simulink model "gm_parallel_prediction_and_cost_function_6phase"  (R2022a)
settings: Solver=FixedStepDiscrete  StartTime=0.0  StopTime=10.0  RelTol=1e-3
undefined symbols (not defined in the file or in its folder): f_c, L_d, L_q, L_x, L_y, p, psi_pm, R_ph
libraries: hdlmdlgenlib x338
(part 5 of 12)

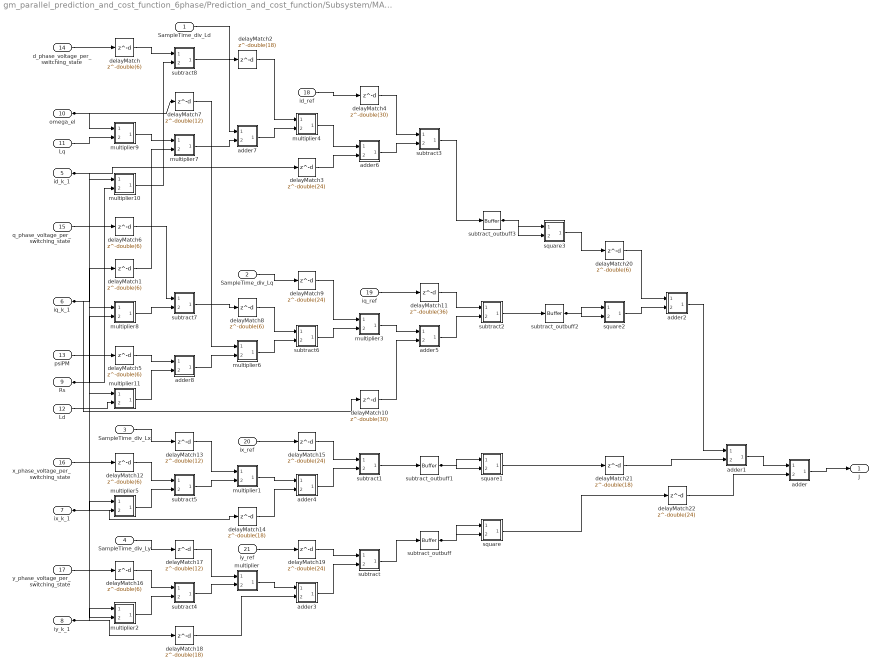
== system gm_parallel_prediction_and_cost_function_6phase/Prediction_and_cost_function/Subsystem/MATLAB Function ==
  SampleTime_div_Ld : Inport  OutDataTypeStr=single  PortDimensions=1  SampleTime=1e-08
  SampleTime_div_Lq : Inport  Port=2  OutDataTypeStr=single  PortDimensions=1  SampleTime=1e-08
  SampleTime_div_Lx : Inport  Port=3  OutDataTypeStr=single  PortDimensions=1  SampleTime=1e-08
  SampleTime_div_Ly : Inport  Port=4  OutDataTypeStr=single  PortDimensions=1  SampleTime=1e-08
  id_k_1 : Inport  Port=5  OutDataTypeStr=single  PortDimensions=1  SampleTime=1e-08
  iq_k_1 : Inport  Port=6  OutDataTypeStr=single  PortDimensions=1  SampleTime=1e-08
  ix_k_1 : Inport  Port=7  OutDataTypeStr=single  PortDimensions=1  SampleTime=1e-08
  iy_k_1 : Inport  Port=8  OutDataTypeStr=single  PortDimensions=1  SampleTime=1e-08
  Rs : Inport  Port=9  OutDataTypeStr=single  PortDimensions=1  SampleTime=1e-08
  omega_el : Inport  Port=10  OutDataTypeStr=single  PortDimensions=1  SampleTime=1e-08
  Lq : Inport  Port=11  OutDataTypeStr=single  PortDimensions=1  SampleTime=1e-08
  Ld : Inport  Port=12  OutDataTypeStr=single  PortDimensions=1  SampleTime=1e-08
  psiPM : Inport  Port=13  OutDataTypeStr=single  PortDimensions=1  SampleTime=1e-08
  d_phase_voltage_per_switching_state : Inport  Port=14  OutDataTypeStr=single  PortDimensions=1  SampleTime=1e-08
  q_phase_voltage_per_switching_state : Inport  Port=15  OutDataTypeStr=single  PortDimensions=1  SampleTime=1e-08
  x_phase_voltage_per_switching_state : Inport  Port=16  OutDataTypeStr=single  PortDimensions=1  SampleTime=1e-08
  y_phase_voltage_per_switching_state : Inport  Port=17  OutDataTypeStr=single  PortDimensions=1  SampleTime=1e-08
  id_ref : Inport  Port=18  OutDataTypeStr=single  PortDimensions=1  SampleTime=1e-08
  iq_ref : Inport  Port=19  OutDataTypeStr=single  PortDimensions=1  SampleTime=1e-08
  ix_ref : Inport  Port=20  OutDataTypeStr=single  PortDimensions=1  SampleTime=1e-08
  iy_ref : Inport  Port=21  OutDataTypeStr=single  PortDimensions=1  SampleTime=1e-08
  adder : Subsystem
      mask Display: disp('NFP\nadd');
  adder1 : Subsystem
      mask Display: disp('NFP\nadd');
  adder2 : Subsystem
      mask Display: disp('NFP\nadd');
  adder3 : Subsystem
      mask Display: disp('NFP\nadd');
  adder4 : Subsystem
      mask Display: disp('NFP\nadd');
  adder5 : Subsystem
      mask Display: disp('NFP\nadd');
  adder6 : Subsystem
      mask Display: disp('NFP\nadd');
  adder7 : Subsystem
      mask Display: disp('NFP\nadd');
  adder8 : Subsystem
      mask Display: disp('NFP\nadd');
  delayMatch{,1,5..6,8,12,16,20} (8 alike) : Delay  DelayLength=double(6)  InitialCondition=0  SampleTime=1e-08
  delayMatch10 : Delay  DelayLength=double(30)  InitialCondition=0  SampleTime=1e-08
  delayMatch11 : Delay  DelayLength=double(36)  InitialCondition=0  SampleTime=1e-08
  delayMatch13 : Delay  DelayLength=double(12)  InitialCondition=0  SampleTime=1e-08
  delayMatch{2,14,18,21} (4 alike) : Delay  DelayLength=double(18)  InitialCondition=0  SampleTime=1e-08
  delayMatch{3,9,15,19,22} (5 alike) : Delay  DelayLength=double(24)  InitialCondition=0  SampleTime=1e-08
  delayMatch17 : Delay  DelayLength=double(12)  InitialCondition=0  SampleTime=1e-08
  delayMatch4 : Delay  DelayLength=double(30)  InitialCondition=0  SampleTime=1e-08
  delayMatch7 : Delay  DelayLength=double(12)  InitialCondition=0  SampleTime=1e-08
  multiplier : Subsystem
      mask Display: disp('NFP\nmul');
  multiplier1 : Subsystem
      mask Display: disp('NFP\nmul');
  multiplier10 : Subsystem
      mask Display: disp('NFP\nmul');
  multiplier11 : Subsystem
      mask Display: disp('NFP\nmul');
  multiplier2 : Subsystem
      mask Display: disp('NFP\nmul');
  multiplier3 : Subsystem
      mask Display: disp('NFP\nmul');
  multiplier4 : Subsystem
      mask Display: disp('NFP\nmul');
  multiplier5 : Subsystem
      mask Display: disp('NFP\nmul');
  multiplier6 : Subsystem
      mask Display: disp('NFP\nmul');
  multiplier7 : Subsystem
      mask Display: disp('NFP\nmul');
  multiplier8 : Subsystem
      mask Display: disp('NFP\nmul');
  multiplier9 : Subsystem
      mask Display: disp('NFP\nmul');
  square : Subsystem
      mask Display: disp('NFP\nmul');
  square1 : Subsystem
      mask Display: disp('NFP\nmul');
  square2 : Subsystem
      mask Display: disp('NFP\nmul');
  square3 : Subsystem
      mask Display: disp('NFP\nmul');
  subtract : Subsystem
      mask Display: disp('NFP\nadd');
  subtract1 : Subsystem
      mask Display: disp('NFP\nadd');
  subtract2 : Subsystem
      mask Display: disp('NFP\nadd');
  subtract3 : Subsystem
      mask Display: disp('NFP\nadd');
  subtract4 : Subsystem
      mask Display: disp('NFP\nadd');
  subtract5 : Subsystem
      mask Display: disp('NFP\nadd');
  subtract6 : Subsystem
      mask Display: disp('NFP\nadd');
  subtract7 : Subsystem
      mask Display: disp('NFP\nadd');
  subtract8 : Subsystem
      mask Display: disp('NFP\nadd');
  subtract_outbuff{,1..3} (4 alike) : hdlmdlgenlib/Buffer
      settings: SourceProductBaseCode=SL
  J : Outport  SampleTime=1e-08  VectorParamsAs1DForOutWhenUnconnected=off
  wires:
  delayMatch2/1 -> multiplier4/1(In1)
  delayMatch9/1 -> multiplier3/1(In1)
  delayMatch13/1 -> multiplier1/1(In1)
  delayMatch17/1 -> multiplier/1(In1)
  delayMatch3/1 -> adder6/2(In2)
  delayMatch1/1 -> multiplier7/2(In2)
  delayMatch14/1 -> adder4/2(In2)
  delayMatch18/1 -> adder3/2(In2)
  delayMatch7/1 -> multiplier6/1(In1)
  delayMatch5/1 -> adder8/1(In1)
  delayMatch/1 -> subtract8/1(In1)
  delayMatch6/1 -> subtract7/1(In1)
  delayMatch12/1 -> subtract5/1(In1)
  delayMatch16/1 -> subtract4/1(In1)
  delayMatch4/1 -> subtract3/1(In1)
  delayMatch11/1 -> subtract2/1(In1)
  delayMatch15/1 -> subtract1/1(In1)
  delayMatch19/1 -> subtract/1(In1)
  delayMatch22/1 -> adder/2(In2)
  subtract_outbuff/1 -> square/2(In2), square/1(In1)
  delayMatch21/1 -> adder1/2(In2)
  subtract_outbuff1/1 -> square1/2(In2), square1/1(In1)
  delayMatch20/1 -> adder2/1(In1)
  subtract_outbuff2/1 -> square2/2(In2), square2/1(In1)
  subtract_outbuff3/1 -> square3/2(In2), square3/1(In1)
  delayMatch8/1 -> subtract6/1(In1)
  adder/1(Out1) -> J/1
  square/1(Out1) -> delayMatch22/1
  adder1/1(Out1) -> adder/1(In1)
  subtract/1(Out1) -> subtract_outbuff/1
  square1/1(Out1) -> delayMatch21/1
  adder2/1(Out1) -> adder1/1(In1)
  adder3/1(Out1) -> subtract/2(In2)
  subtract1/1(Out1) -> subtract_outbuff1/1
  square2/1(Out1) -> adder2/2(In2)
  square3/1(Out1) -> delayMatch20/1
  multiplier/1(Out1) -> adder3/1(In1)
  adder4/1(Out1) -> subtract1/2(In2)
  subtract2/1(Out1) -> subtract_outbuff2/1
  subtract3/1(Out1) -> subtract_outbuff3/1
  subtract4/1(Out1) -> multiplier/2(In2)
  multiplier1/1(Out1) -> adder4/1(In1)
  adder5/1(Out1) -> subtract2/2(In2)
  adder6/1(Out1) -> subtract3/2(In2)
  multiplier2/1(Out1) -> subtract4/2(In2)
  subtract5/1(Out1) -> multiplier1/2(In2)
  multiplier3/1(Out1) -> adder5/1(In1)
  multiplier4/1(Out1) -> adder6/1(In1)
  multiplier5/1(Out1) -> subtract5/2(In2)
  subtract6/1(Out1) -> multiplier3/2(In2)
  adder7/1(Out1) -> multiplier4/2(In2)
  multiplier6/1(Out1) -> subtract6/2(In2)
  subtract7/1(Out1) -> delayMatch8/1
  multiplier7/1(Out1) -> adder7/2(In2)
  subtract8/1(Out1) -> adder7/1(In1)
  adder8/1(Out1) -> multiplier6/2(In2)
  multiplier8/1(Out1) -> subtract7/2(In2)
  multiplier9/1(Out1) -> multiplier7/1(In1)
  multiplier10/1(Out1) -> subtract8/2(In2)
  multiplier11/1(Out1) -> adder8/2(In2)
  delayMatch10/1 -> adder5/2(In2)
  SampleTime_div_Ld/1 -> delayMatch2/1
  SampleTime_div_Lq/1 -> delayMatch9/1
  SampleTime_div_Lx/1 -> delayMatch13/1
  SampleTime_div_Ly/1 -> delayMatch17/1
  id_k_1/1 -> delayMatch3/1, multiplier11/1(In1), multiplier10/1(In1)
  iq_k_1/1 -> delayMatch10/1, delayMatch1/1, multiplier8/1(In1)
  ix_k_1/1 -> delayMatch14/1, multiplier5/1(In1)
  iy_k_1/1 -> delayMatch18/1, multiplier2/1(In1)
  Rs/1 -> multiplier10/2(In2), multiplier8/2(In2), multiplier5/2(In2), multiplier2/2(In2)
  omega_el/1 -> delayMatch7/1, multiplier9/1(In1)
  Lq/1 -> multiplier9/2(In2)
  Ld/1 -> multiplier11/2(In2)
  psiPM/1 -> delayMatch5/1
  d_phase_voltage_per_switching_state/1 -> delayMatch/1
  q_phase_voltage_per_switching_state/1 -> delayMatch6/1
  x_phase_voltage_per_switching_state/1 -> delayMatch12/1
  y_phase_voltage_per_switching_state/1 -> delayMatch16/1
  id_ref/1 -> delayMatch4/1
  iq_ref/1 -> delayMatch11/1
  ix_ref/1 -> delayMatch15/1
  iy_ref/1 -> delayMatch19/1

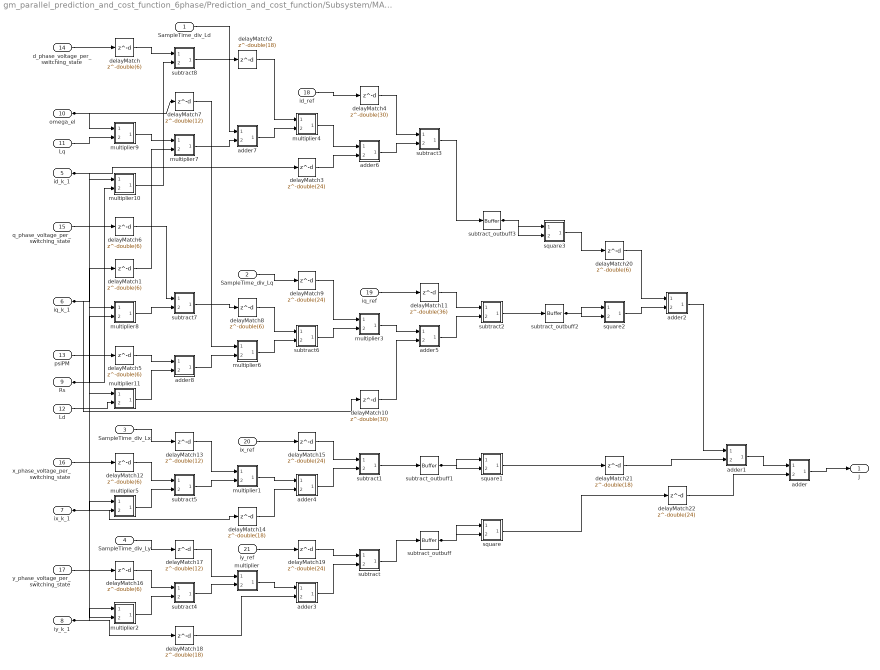
== system gm_parallel_prediction_and_cost_function_6phase/Prediction_and_cost_function/Subsystem/MATLAB Function1 ==
  SampleTime_div_Ld : Inport  OutDataTypeStr=single  PortDimensions=1  SampleTime=1e-08
  SampleTime_div_Lq : Inport  Port=2  OutDataTypeStr=single  PortDimensions=1  SampleTime=1e-08
  SampleTime_div_Lx : Inport  Port=3  OutDataTypeStr=single  PortDimensions=1  SampleTime=1e-08
  SampleTime_div_Ly : Inport  Port=4  OutDataTypeStr=single  PortDimensions=1  SampleTime=1e-08
  id_k_1 : Inport  Port=5  OutDataTypeStr=single  PortDimensions=1  SampleTime=1e-08
  iq_k_1 : Inport  Port=6  OutDataTypeStr=single  PortDimensions=1  SampleTime=1e-08
  ix_k_1 : Inport  Port=7  OutDataTypeStr=single  PortDimensions=1  SampleTime=1e-08
  iy_k_1 : Inport  Port=8  OutDataTypeStr=single  PortDimensions=1  SampleTime=1e-08
  Rs : Inport  Port=9  OutDataTypeStr=single  PortDimensions=1  SampleTime=1e-08
  omega_el : Inport  Port=10  OutDataTypeStr=single  PortDimensions=1  SampleTime=1e-08
  Lq : Inport  Port=11  OutDataTypeStr=single  PortDimensions=1  SampleTime=1e-08
  Ld : Inport  Port=12  OutDataTypeStr=single  PortDimensions=1  SampleTime=1e-08
  psiPM : Inport  Port=13  OutDataTypeStr=single  PortDimensions=1  SampleTime=1e-08
  d_phase_voltage_per_switching_state : Inport  Port=14  OutDataTypeStr=single  PortDimensions=1  SampleTime=1e-08
  q_phase_voltage_per_switching_state : Inport  Port=15  OutDataTypeStr=single  PortDimensions=1  SampleTime=1e-08
  x_phase_voltage_per_switching_state : Inport  Port=16  OutDataTypeStr=single  PortDimensions=1  SampleTime=1e-08
  y_phase_voltage_per_switching_state : Inport  Port=17  OutDataTypeStr=single  PortDimensions=1  SampleTime=1e-08
  id_ref : Inport  Port=18  OutDataTypeStr=single  PortDimensions=1  SampleTime=1e-08
  iq_ref : Inport  Port=19  OutDataTypeStr=single  PortDimensions=1  SampleTime=1e-08
  ix_ref : Inport  Port=20  OutDataTypeStr=single  PortDimensions=1  SampleTime=1e-08
  iy_ref : Inport  Port=21  OutDataTypeStr=single  PortDimensions=1  SampleTime=1e-08
  adder : Subsystem
      mask Display: disp('NFP\nadd');
  adder1 : Subsystem
      mask Display: disp('NFP\nadd');
  adder2 : Subsystem
      mask Display: disp('NFP\nadd');
  adder3 : Subsystem
      mask Display: disp('NFP\nadd');
  adder4 : Subsystem
      mask Display: disp('NFP\nadd');
  adder5 : Subsystem
      mask Display: disp('NFP\nadd');
  adder6 : Subsystem
      mask Display: disp('NFP\nadd');
  adder7 : Subsystem
      mask Display: disp('NFP\nadd');
  adder8 : Subsystem
      mask Display: disp('NFP\nadd');
  delayMatch{,1,5..6,8,12,16,20} (8 alike) : Delay  DelayLength=double(6)  InitialCondition=0  SampleTime=1e-08
  delayMatch10 : Delay  DelayLength=double(30)  InitialCondition=0  SampleTime=1e-08
  delayMatch11 : Delay  DelayLength=double(36)  InitialCondition=0  SampleTime=1e-08
  delayMatch13 : Delay  DelayLength=double(12)  InitialCondition=0  SampleTime=1e-08
  delayMatch{2,14,18,21} (4 alike) : Delay  DelayLength=double(18)  InitialCondition=0  SampleTime=1e-08
  delayMatch{3,9,15,19,22} (5 alike) : Delay  DelayLength=double(24)  InitialCondition=0  SampleTime=1e-08
  delayMatch17 : Delay  DelayLength=double(12)  InitialCondition=0  SampleTime=1e-08
  delayMatch4 : Delay  DelayLength=double(30)  InitialCondition=0  SampleTime=1e-08
  delayMatch7 : Delay  DelayLength=double(12)  InitialCondition=0  SampleTime=1e-08
  multiplier : Subsystem
      mask Display: disp('NFP\nmul');
  multiplier1 : Subsystem
      mask Display: disp('NFP\nmul');
  multiplier10 : Subsystem
      mask Display: disp('NFP\nmul');
  multiplier11 : Subsystem
      mask Display: disp('NFP\nmul');
  multiplier2 : Subsystem
      mask Display: disp('NFP\nmul');
  multiplier3 : Subsystem
      mask Display: disp('NFP\nmul');
  multiplier4 : Subsystem
      mask Display: disp('NFP\nmul');
  multiplier5 : Subsystem
      mask Display: disp('NFP\nmul');
  multiplier6 : Subsystem
      mask Display: disp('NFP\nmul');
  multiplier7 : Subsystem
      mask Display: disp('NFP\nmul');
  multiplier8 : Subsystem
      mask Display: disp('NFP\nmul');
  multiplier9 : Subsystem
      mask Display: disp('NFP\nmul');
  square : Subsystem
      mask Display: disp('NFP\nmul');
  square1 : Subsystem
      mask Display: disp('NFP\nmul');
  square2 : Subsystem
      mask Display: disp('NFP\nmul');
  square3 : Subsystem
      mask Display: disp('NFP\nmul');
  subtract : Subsystem
      mask Display: disp('NFP\nadd');
  subtract1 : Subsystem
      mask Display: disp('NFP\nadd');
  subtract2 : Subsystem
      mask Display: disp('NFP\nadd');
  subtract3 : Subsystem
      mask Display: disp('NFP\nadd');
  subtract4 : Subsystem
      mask Display: disp('NFP\nadd');
  subtract5 : Subsystem
      mask Display: disp('NFP\nadd');
  subtract6 : Subsystem
      mask Display: disp('NFP\nadd');
  subtract7 : Subsystem
      mask Display: disp('NFP\nadd');
  subtract8 : Subsystem
      mask Display: disp('NFP\nadd');
  subtract_outbuff{,1..3} (4 alike) : hdlmdlgenlib/Buffer
      settings: SourceProductBaseCode=SL
  J : Outport  SampleTime=1e-08  VectorParamsAs1DForOutWhenUnconnected=off
  wires:
  iy_ref/1 -> delayMatch19/1
  ix_ref/1 -> delayMatch15/1
  iq_ref/1 -> delayMatch11/1
  id_ref/1 -> delayMatch4/1
  y_phase_voltage_per_switching_state/1 -> delayMatch16/1
  x_phase_voltage_per_switching_state/1 -> delayMatch12/1
  q_phase_voltage_per_switching_state/1 -> delayMatch6/1
  d_phase_voltage_per_switching_state/1 -> delayMatch/1
  psiPM/1 -> delayMatch5/1
  Ld/1 -> multiplier11/2(In2)
  Lq/1 -> multiplier9/2(In2)
  omega_el/1 -> multiplier9/1(In1), delayMatch7/1
  Rs/1 -> multiplier2/2(In2), multiplier5/2(In2), multiplier8/2(In2), multiplier10/2(In2)
  iy_k_1/1 -> multiplier2/1(In1), delayMatch18/1
  ix_k_1/1 -> multiplier5/1(In1), delayMatch14/1
  iq_k_1/1 -> multiplier8/1(In1), delayMatch1/1, delayMatch10/1
  id_k_1/1 -> multiplier10/1(In1), multiplier11/1(In1), delayMatch3/1
  SampleTime_div_Ly/1 -> delayMatch17/1
  SampleTime_div_Lx/1 -> delayMatch13/1
  SampleTime_div_Lq/1 -> delayMatch9/1
  SampleTime_div_Ld/1 -> delayMatch2/1
  delayMatch10/1 -> adder5/2(In2)
  multiplier11/1(Out1) -> adder8/2(In2)
  multiplier10/1(Out1) -> subtract8/2(In2)
  multiplier9/1(Out1) -> multiplier7/1(In1)
  multiplier8/1(Out1) -> subtract7/2(In2)
  adder8/1(Out1) -> multiplier6/2(In2)
  subtract8/1(Out1) -> adder7/1(In1)
  multiplier7/1(Out1) -> adder7/2(In2)
  subtract7/1(Out1) -> delayMatch8/1
  multiplier6/1(Out1) -> subtract6/2(In2)
  adder7/1(Out1) -> multiplier4/2(In2)
  subtract6/1(Out1) -> multiplier3/2(In2)
  multiplier5/1(Out1) -> subtract5/2(In2)
  multiplier4/1(Out1) -> adder6/1(In1)
  multiplier3/1(Out1) -> adder5/1(In1)
  subtract5/1(Out1) -> multiplier1/2(In2)
  multiplier2/1(Out1) -> subtract4/2(In2)
  adder6/1(Out1) -> subtract3/2(In2)
  adder5/1(Out1) -> subtract2/2(In2)
  multiplier1/1(Out1) -> adder4/1(In1)
  subtract4/1(Out1) -> multiplier/2(In2)
  subtract3/1(Out1) -> subtract_outbuff3/1
  subtract2/1(Out1) -> subtract_outbuff2/1
  adder4/1(Out1) -> subtract1/2(In2)
  multiplier/1(Out1) -> adder3/1(In1)
  square3/1(Out1) -> delayMatch20/1
  square2/1(Out1) -> adder2/2(In2)
  subtract1/1(Out1) -> subtract_outbuff1/1
  adder3/1(Out1) -> subtract/2(In2)
  adder2/1(Out1) -> adder1/1(In1)
  square1/1(Out1) -> delayMatch21/1
  subtract/1(Out1) -> subtract_outbuff/1
  adder1/1(Out1) -> adder/1(In1)
  square/1(Out1) -> delayMatch22/1
  adder/1(Out1) -> J/1
  delayMatch8/1 -> subtract6/1(In1)
  subtract_outbuff3/1 -> square3/1(In1), square3/2(In2)
  subtract_outbuff2/1 -> square2/1(In1), square2/2(In2)
  delayMatch20/1 -> adder2/1(In1)
  subtract_outbuff1/1 -> square1/1(In1), square1/2(In2)
  delayMatch21/1 -> adder1/2(In2)
  subtract_outbuff/1 -> square/1(In1), square/2(In2)
  delayMatch22/1 -> adder/2(In2)
  delayMatch19/1 -> subtract/1(In1)
  delayMatch15/1 -> subtract1/1(In1)
  delayMatch11/1 -> subtract2/1(In1)
  delayMatch4/1 -> subtract3/1(In1)
  delayMatch16/1 -> subtract4/1(In1)
  delayMatch12/1 -> subtract5/1(In1)
  delayMatch6/1 -> subtract7/1(In1)
  delayMatch/1 -> subtract8/1(In1)
  delayMatch5/1 -> adder8/1(In1)
  delayMatch7/1 -> multiplier6/1(In1)
  delayMatch18/1 -> adder3/2(In2)
  delayMatch14/1 -> adder4/2(In2)
  delayMatch1/1 -> multiplier7/2(In2)
  delayMatch3/1 -> adder6/2(In2)
  delayMatch17/1 -> multiplier/1(In1)
  delayMatch13/1 -> multiplier1/1(In1)
  delayMatch9/1 -> multiplier3/1(In1)
  delayMatch2/1 -> multiplier4/1(In1)

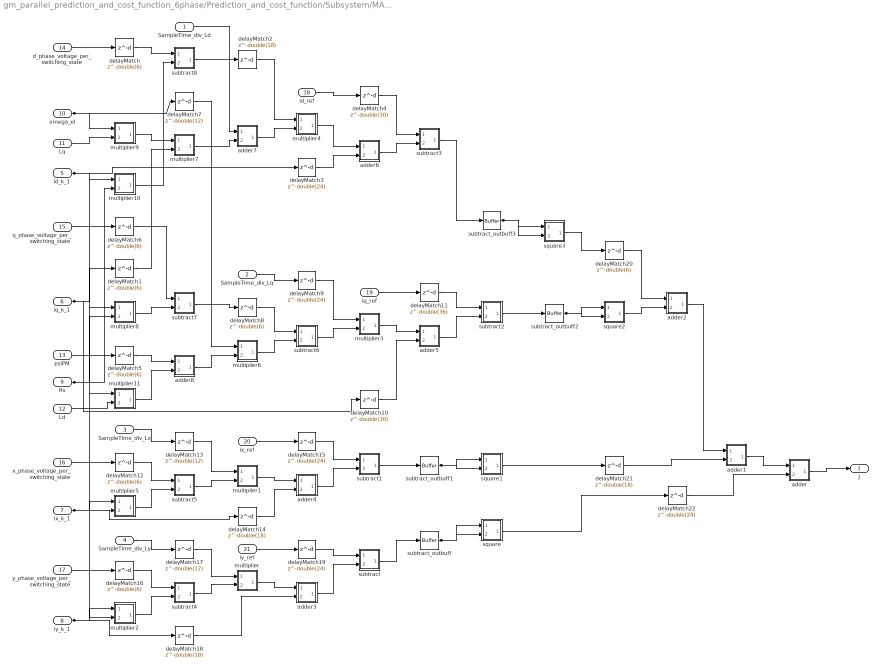
== system gm_parallel_prediction_and_cost_function_6phase/Prediction_and_cost_function/Subsystem/MATLAB Function10 ==
  SampleTime_div_Ld : Inport  OutDataTypeStr=single  PortDimensions=1  SampleTime=1e-08
  SampleTime_div_Lq : Inport  Port=2  OutDataTypeStr=single  PortDimensions=1  SampleTime=1e-08
  SampleTime_div_Lx : Inport  Port=3  OutDataTypeStr=single  PortDimensions=1  SampleTime=1e-08
  SampleTime_div_Ly : Inport  Port=4  OutDataTypeStr=single  PortDimensions=1  SampleTime=1e-08
  id_k_1 : Inport  Port=5  OutDataTypeStr=single  PortDimensions=1  SampleTime=1e-08
  iq_k_1 : Inport  Port=6  OutDataTypeStr=single  PortDimensions=1  SampleTime=1e-08
  ix_k_1 : Inport  Port=7  OutDataTypeStr=single  PortDimensions=1  SampleTime=1e-08
  iy_k_1 : Inport  Port=8  OutDataTypeStr=single  PortDimensions=1  SampleTime=1e-08
  Rs : Inport  Port=9  OutDataTypeStr=single  PortDimensions=1  SampleTime=1e-08
  omega_el : Inport  Port=10  OutDataTypeStr=single  PortDimensions=1  SampleTime=1e-08
  Lq : Inport  Port=11  OutDataTypeStr=single  PortDimensions=1  SampleTime=1e-08
  Ld : Inport  Port=12  OutDataTypeStr=single  PortDimensions=1  SampleTime=1e-08
  psiPM : Inport  Port=13  OutDataTypeStr=single  PortDimensions=1  SampleTime=1e-08
  d_phase_voltage_per_switching_state : Inport  Port=14  OutDataTypeStr=single  PortDimensions=1  SampleTime=1e-08
  q_phase_voltage_per_switching_state : Inport  Port=15  OutDataTypeStr=single  PortDimensions=1  SampleTime=1e-08
  x_phase_voltage_per_switching_state : Inport  Port=16  OutDataTypeStr=single  PortDimensions=1  SampleTime=1e-08
  y_phase_voltage_per_switching_state : Inport  Port=17  OutDataTypeStr=single  PortDimensions=1  SampleTime=1e-08
  id_ref : Inport  Port=18  OutDataTypeStr=single  PortDimensions=1  SampleTime=1e-08
  iq_ref : Inport  Port=19  OutDataTypeStr=single  PortDimensions=1  SampleTime=1e-08
  ix_ref : Inport  Port=20  OutDataTypeStr=single  PortDimensions=1  SampleTime=1e-08
  iy_ref : Inport  Port=21  OutDataTypeStr=single  PortDimensions=1  SampleTime=1e-08
  adder : Subsystem
      mask Display: disp('NFP\nadd');
  adder1 : Subsystem
      mask Display: disp('NFP\nadd');
  adder2 : Subsystem
      mask Display: disp('NFP\nadd');
  adder3 : Subsystem
      mask Display: disp('NFP\nadd');
  adder4 : Subsystem
      mask Display: disp('NFP\nadd');
  adder5 : Subsystem
      mask Display: disp('NFP\nadd');
  adder6 : Subsystem
      mask Display: disp('NFP\nadd');
  adder7 : Subsystem
      mask Display: disp('NFP\nadd');
  adder8 : Subsystem
      mask Display: disp('NFP\nadd');
  delayMatch{,1,5..6,8,12,16,20} (8 alike) : Delay  DelayLength=double(6)  InitialCondition=0  SampleTime=1e-08
  delayMatch10 : Delay  DelayLength=double(30)  InitialCondition=0  SampleTime=1e-08
  delayMatch11 : Delay  DelayLength=double(36)  InitialCondition=0  SampleTime=1e-08
  delayMatch13 : Delay  DelayLength=double(12)  InitialCondition=0  SampleTime=1e-08
  delayMatch{2,14,18,21} (4 alike) : Delay  DelayLength=double(18)  InitialCondition=0  SampleTime=1e-08
  delayMatch{3,9,15,19,22} (5 alike) : Delay  DelayLength=double(24)  InitialCondition=0  SampleTime=1e-08
  delayMatch17 : Delay  DelayLength=double(12)  InitialCondition=0  SampleTime=1e-08
  delayMatch4 : Delay  DelayLength=double(30)  InitialCondition=0  SampleTime=1e-08
  delayMatch7 : Delay  DelayLength=double(12)  InitialCondition=0  SampleTime=1e-08
  multiplier : Subsystem
      mask Display: disp('NFP\nmul');
  multiplier1 : Subsystem
      mask Display: disp('NFP\nmul');
  multiplier10 : Subsystem
      mask Display: disp('NFP\nmul');
  multiplier11 : Subsystem
      mask Display: disp('NFP\nmul');
  multiplier2 : Subsystem
      mask Display: disp('NFP\nmul');
  multiplier3 : Subsystem
      mask Display: disp('NFP\nmul');
  multiplier4 : Subsystem
      mask Display: disp('NFP\nmul');
  multiplier5 : Subsystem
      mask Display: disp('NFP\nmul');
  multiplier6 : Subsystem
      mask Display: disp('NFP\nmul');
  multiplier7 : Subsystem
      mask Display: disp('NFP\nmul');
  multiplier8 : Subsystem
      mask Display: disp('NFP\nmul');
  multiplier9 : Subsystem
      mask Display: disp('NFP\nmul');
  square : Subsystem
      mask Display: disp('NFP\nmul');
  square1 : Subsystem
      mask Display: disp('NFP\nmul');
  square2 : Subsystem
      mask Display: disp('NFP\nmul');
  square3 : Subsystem
      mask Display: disp('NFP\nmul');
  subtract : Subsystem
      mask Display: disp('NFP\nadd');
  subtract1 : Subsystem
      mask Display: disp('NFP\nadd');
  subtract2 : Subsystem
      mask Display: disp('NFP\nadd');
  subtract3 : Subsystem
      mask Display: disp('NFP\nadd');
  subtract4 : Subsystem
      mask Display: disp('NFP\nadd');
  subtract5 : Subsystem
      mask Display: disp('NFP\nadd');
  subtract6 : Subsystem
      mask Display: disp('NFP\nadd');
  subtract7 : Subsystem
      mask Display: disp('NFP\nadd');
  subtract8 : Subsystem
      mask Display: disp('NFP\nadd');
  subtract_outbuff{,1..3} (4 alike) : hdlmdlgenlib/Buffer
      settings: SourceProductBaseCode=SL
  J : Outport  SampleTime=1e-08  VectorParamsAs1DForOutWhenUnconnected=off
  wires:
  iy_ref/1 -> delayMatch19/1
  ix_ref/1 -> delayMatch15/1
  iq_ref/1 -> delayMatch11/1
  id_ref/1 -> delayMatch4/1
  y_phase_voltage_per_switching_state/1 -> delayMatch16/1
  x_phase_voltage_per_switching_state/1 -> delayMatch12/1
  q_phase_voltage_per_switching_state/1 -> delayMatch6/1
  d_phase_voltage_per_switching_state/1 -> delayMatch/1
  psiPM/1 -> delayMatch5/1
  Ld/1 -> multiplier11/2(In2)
  Lq/1 -> multiplier9/2(In2)
  omega_el/1 -> multiplier9/1(In1), delayMatch7/1
  Rs/1 -> multiplier2/2(In2), multiplier5/2(In2), multiplier8/2(In2), multiplier10/2(In2)
  iy_k_1/1 -> multiplier2/1(In1), delayMatch18/1
  ix_k_1/1 -> multiplier5/1(In1), delayMatch14/1
  iq_k_1/1 -> multiplier8/1(In1), delayMatch1/1, delayMatch10/1
  id_k_1/1 -> multiplier10/1(In1), multiplier11/1(In1), delayMatch3/1
  SampleTime_div_Ly/1 -> delayMatch17/1
  SampleTime_div_Lx/1 -> delayMatch13/1
  SampleTime_div_Lq/1 -> delayMatch9/1
  SampleTime_div_Ld/1 -> delayMatch2/1
  delayMatch10/1 -> adder5/2(In2)
  multiplier11/1(Out1) -> adder8/2(In2)
  multiplier10/1(Out1) -> subtract8/2(In2)
  multiplier9/1(Out1) -> multiplier7/1(In1)
  multiplier8/1(Out1) -> subtract7/2(In2)
  adder8/1(Out1) -> multiplier6/2(In2)
  subtract8/1(Out1) -> adder7/1(In1)
  multiplier7/1(Out1) -> adder7/2(In2)
  subtract7/1(Out1) -> delayMatch8/1
  multiplier6/1(Out1) -> subtract6/2(In2)
  adder7/1(Out1) -> multiplier4/2(In2)
  subtract6/1(Out1) -> multiplier3/2(In2)
  multiplier5/1(Out1) -> subtract5/2(In2)
  multiplier4/1(Out1) -> adder6/1(In1)
  multiplier3/1(Out1) -> adder5/1(In1)
  subtract5/1(Out1) -> multiplier1/2(In2)
  multiplier2/1(Out1) -> subtract4/2(In2)
  adder6/1(Out1) -> subtract3/2(In2)
  adder5/1(Out1) -> subtract2/2(In2)
  multiplier1/1(Out1) -> adder4/1(In1)
  subtract4/1(Out1) -> multiplier/2(In2)
  subtract3/1(Out1) -> subtract_outbuff3/1
  subtract2/1(Out1) -> subtract_outbuff2/1
  adder4/1(Out1) -> subtract1/2(In2)
  multiplier/1(Out1) -> adder3/1(In1)
  square3/1(Out1) -> delayMatch20/1
  square2/1(Out1) -> adder2/2(In2)
  subtract1/1(Out1) -> subtract_outbuff1/1
  adder3/1(Out1) -> subtract/2(In2)
  adder2/1(Out1) -> adder1/1(In1)
  square1/1(Out1) -> delayMatch21/1
  subtract/1(Out1) -> subtract_outbuff/1
  adder1/1(Out1) -> adder/1(In1)
  square/1(Out1) -> delayMatch22/1
  adder/1(Out1) -> J/1
  delayMatch8/1 -> subtract6/1(In1)
  subtract_outbuff3/1 -> square3/1(In1), square3/2(In2)
  subtract_outbuff2/1 -> square2/1(In1), square2/2(In2)
  delayMatch20/1 -> adder2/1(In1)
  subtract_outbuff1/1 -> square1/1(In1), square1/2(In2)
  delayMatch21/1 -> adder1/2(In2)
  subtract_outbuff/1 -> square/1(In1), square/2(In2)
  delayMatch22/1 -> adder/2(In2)
  delayMatch19/1 -> subtract/1(In1)
  delayMatch15/1 -> subtract1/1(In1)
  delayMatch11/1 -> subtract2/1(In1)
  delayMatch4/1 -> subtract3/1(In1)
  delayMatch16/1 -> subtract4/1(In1)
  delayMatch12/1 -> subtract5/1(In1)
  delayMatch6/1 -> subtract7/1(In1)
  delayMatch/1 -> subtract8/1(In1)
  delayMatch5/1 -> adder8/1(In1)
  delayMatch7/1 -> multiplier6/1(In1)
  delayMatch18/1 -> adder3/2(In2)
  delayMatch14/1 -> adder4/2(In2)
  delayMatch1/1 -> multiplier7/2(In2)
  delayMatch3/1 -> adder6/2(In2)
  delayMatch17/1 -> multiplier/1(In1)
  delayMatch13/1 -> multiplier1/1(In1)
  delayMatch9/1 -> multiplier3/1(In1)
  delayMatch2/1 -> multiplier4/1(In1)

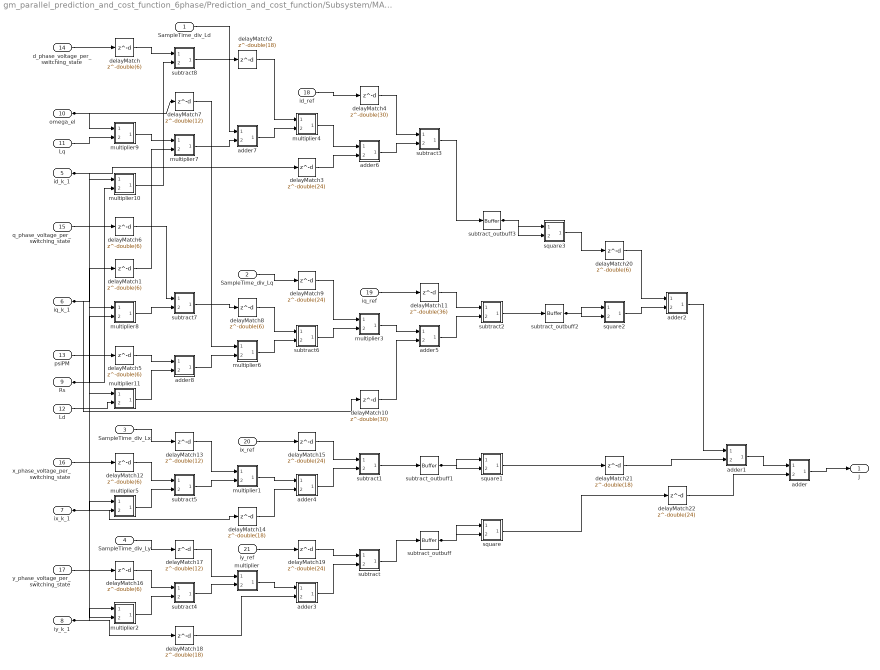
== system gm_parallel_prediction_and_cost_function_6phase/Prediction_and_cost_function/Subsystem/MATLAB Function11 ==
  SampleTime_div_Ld : Inport  OutDataTypeStr=single  PortDimensions=1  SampleTime=1e-08
  SampleTime_div_Lq : Inport  Port=2  OutDataTypeStr=single  PortDimensions=1  SampleTime=1e-08
  SampleTime_div_Lx : Inport  Port=3  OutDataTypeStr=single  PortDimensions=1  SampleTime=1e-08
  SampleTime_div_Ly : Inport  Port=4  OutDataTypeStr=single  PortDimensions=1  SampleTime=1e-08
  id_k_1 : Inport  Port=5  OutDataTypeStr=single  PortDimensions=1  SampleTime=1e-08
  iq_k_1 : Inport  Port=6  OutDataTypeStr=single  PortDimensions=1  SampleTime=1e-08
  ix_k_1 : Inport  Port=7  OutDataTypeStr=single  PortDimensions=1  SampleTime=1e-08
  iy_k_1 : Inport  Port=8  OutDataTypeStr=single  PortDimensions=1  SampleTime=1e-08
  Rs : Inport  Port=9  OutDataTypeStr=single  PortDimensions=1  SampleTime=1e-08
  omega_el : Inport  Port=10  OutDataTypeStr=single  PortDimensions=1  SampleTime=1e-08
  Lq : Inport  Port=11  OutDataTypeStr=single  PortDimensions=1  SampleTime=1e-08
  Ld : Inport  Port=12  OutDataTypeStr=single  PortDimensions=1  SampleTime=1e-08
  psiPM : Inport  Port=13  OutDataTypeStr=single  PortDimensions=1  SampleTime=1e-08
  d_phase_voltage_per_switching_state : Inport  Port=14  OutDataTypeStr=single  PortDimensions=1  SampleTime=1e-08
  q_phase_voltage_per_switching_state : Inport  Port=15  OutDataTypeStr=single  PortDimensions=1  SampleTime=1e-08
  x_phase_voltage_per_switching_state : Inport  Port=16  OutDataTypeStr=single  PortDimensions=1  SampleTime=1e-08
  y_phase_voltage_per_switching_state : Inport  Port=17  OutDataTypeStr=single  PortDimensions=1  SampleTime=1e-08
  id_ref : Inport  Port=18  OutDataTypeStr=single  PortDimensions=1  SampleTime=1e-08
  iq_ref : Inport  Port=19  OutDataTypeStr=single  PortDimensions=1  SampleTime=1e-08
  ix_ref : Inport  Port=20  OutDataTypeStr=single  PortDimensions=1  SampleTime=1e-08
  iy_ref : Inport  Port=21  OutDataTypeStr=single  PortDimensions=1  SampleTime=1e-08
  adder : Subsystem
      mask Display: disp('NFP\nadd');
  adder1 : Subsystem
      mask Display: disp('NFP\nadd');
  adder2 : Subsystem
      mask Display: disp('NFP\nadd');
  adder3 : Subsystem
      mask Display: disp('NFP\nadd');
  adder4 : Subsystem
      mask Display: disp('NFP\nadd');
  adder5 : Subsystem
      mask Display: disp('NFP\nadd');
  adder6 : Subsystem
      mask Display: disp('NFP\nadd');
  adder7 : Subsystem
      mask Display: disp('NFP\nadd');
  adder8 : Subsystem
      mask Display: disp('NFP\nadd');
  delayMatch{,1,5..6,8,12,16,20} (8 alike) : Delay  DelayLength=double(6)  InitialCondition=0  SampleTime=1e-08
  delayMatch10 : Delay  DelayLength=double(30)  InitialCondition=0  SampleTime=1e-08
  delayMatch11 : Delay  DelayLength=double(36)  InitialCondition=0  SampleTime=1e-08
  delayMatch13 : Delay  DelayLength=double(12)  InitialCondition=0  SampleTime=1e-08
  delayMatch{2,14,18,21} (4 alike) : Delay  DelayLength=double(18)  InitialCondition=0  SampleTime=1e-08
  delayMatch{3,9,15,19,22} (5 alike) : Delay  DelayLength=double(24)  InitialCondition=0  SampleTime=1e-08
  delayMatch17 : Delay  DelayLength=double(12)  InitialCondition=0  SampleTime=1e-08
  delayMatch4 : Delay  DelayLength=double(30)  InitialCondition=0  SampleTime=1e-08
  delayMatch7 : Delay  DelayLength=double(12)  InitialCondition=0  SampleTime=1e-08
  multiplier : Subsystem
      mask Display: disp('NFP\nmul');
  multiplier1 : Subsystem
      mask Display: disp('NFP\nmul');
  multiplier10 : Subsystem
      mask Display: disp('NFP\nmul');
  multiplier11 : Subsystem
      mask Display: disp('NFP\nmul');
  multiplier2 : Subsystem
      mask Display: disp('NFP\nmul');
  multiplier3 : Subsystem
      mask Display: disp('NFP\nmul');
  multiplier4 : Subsystem
      mask Display: disp('NFP\nmul');
  multiplier5 : Subsystem
      mask Display: disp('NFP\nmul');
  multiplier6 : Subsystem
      mask Display: disp('NFP\nmul');
  multiplier7 : Subsystem
      mask Display: disp('NFP\nmul');
  multiplier8 : Subsystem
      mask Display: disp('NFP\nmul');
  multiplier9 : Subsystem
      mask Display: disp('NFP\nmul');
  square : Subsystem
      mask Display: disp('NFP\nmul');
  square1 : Subsystem
      mask Display: disp('NFP\nmul');
  square2 : Subsystem
      mask Display: disp('NFP\nmul');
  square3 : Subsystem
      mask Display: disp('NFP\nmul');
  subtract : Subsystem
      mask Display: disp('NFP\nadd');
  subtract1 : Subsystem
      mask Display: disp('NFP\nadd');
  subtract2 : Subsystem
      mask Display: disp('NFP\nadd');
  subtract3 : Subsystem
      mask Display: disp('NFP\nadd');
  subtract4 : Subsystem
      mask Display: disp('NFP\nadd');
  subtract5 : Subsystem
      mask Display: disp('NFP\nadd');
  subtract6 : Subsystem
      mask Display: disp('NFP\nadd');
  subtract7 : Subsystem
      mask Display: disp('NFP\nadd');
  subtract8 : Subsystem
      mask Display: disp('NFP\nadd');
  subtract_outbuff{,1..3} (4 alike) : hdlmdlgenlib/Buffer
      settings: SourceProductBaseCode=SL
  J : Outport  SampleTime=1e-08  VectorParamsAs1DForOutWhenUnconnected=off
  wires:
  iy_ref/1 -> delayMatch19/1
  ix_ref/1 -> delayMatch15/1
  iq_ref/1 -> delayMatch11/1
  id_ref/1 -> delayMatch4/1
  y_phase_voltage_per_switching_state/1 -> delayMatch16/1
  x_phase_voltage_per_switching_state/1 -> delayMatch12/1
  q_phase_voltage_per_switching_state/1 -> delayMatch6/1
  d_phase_voltage_per_switching_state/1 -> delayMatch/1
  psiPM/1 -> delayMatch5/1
  Ld/1 -> multiplier11/2(In2)
  Lq/1 -> multiplier9/2(In2)
  omega_el/1 -> multiplier9/1(In1), delayMatch7/1
  Rs/1 -> multiplier2/2(In2), multiplier5/2(In2), multiplier8/2(In2), multiplier10/2(In2)
  iy_k_1/1 -> multiplier2/1(In1), delayMatch18/1
  ix_k_1/1 -> multiplier5/1(In1), delayMatch14/1
  iq_k_1/1 -> multiplier8/1(In1), delayMatch1/1, delayMatch10/1
  id_k_1/1 -> multiplier10/1(In1), multiplier11/1(In1), delayMatch3/1
  SampleTime_div_Ly/1 -> delayMatch17/1
  SampleTime_div_Lx/1 -> delayMatch13/1
  SampleTime_div_Lq/1 -> delayMatch9/1
  SampleTime_div_Ld/1 -> delayMatch2/1
  delayMatch10/1 -> adder5/2(In2)
  multiplier11/1(Out1) -> adder8/2(In2)
  multiplier10/1(Out1) -> subtract8/2(In2)
  multiplier9/1(Out1) -> multiplier7/1(In1)
  multiplier8/1(Out1) -> subtract7/2(In2)
  adder8/1(Out1) -> multiplier6/2(In2)
  subtract8/1(Out1) -> adder7/1(In1)
  multiplier7/1(Out1) -> adder7/2(In2)
  subtract7/1(Out1) -> delayMatch8/1
  multiplier6/1(Out1) -> subtract6/2(In2)
  adder7/1(Out1) -> multiplier4/2(In2)
  subtract6/1(Out1) -> multiplier3/2(In2)
  multiplier5/1(Out1) -> subtract5/2(In2)
  multiplier4/1(Out1) -> adder6/1(In1)
  multiplier3/1(Out1) -> adder5/1(In1)
  subtract5/1(Out1) -> multiplier1/2(In2)
  multiplier2/1(Out1) -> subtract4/2(In2)
  adder6/1(Out1) -> subtract3/2(In2)
  adder5/1(Out1) -> subtract2/2(In2)
  multiplier1/1(Out1) -> adder4/1(In1)
  subtract4/1(Out1) -> multiplier/2(In2)
  subtract3/1(Out1) -> subtract_outbuff3/1
  subtract2/1(Out1) -> subtract_outbuff2/1
  adder4/1(Out1) -> subtract1/2(In2)
  multiplier/1(Out1) -> adder3/1(In1)
  square3/1(Out1) -> delayMatch20/1
  square2/1(Out1) -> adder2/2(In2)
  subtract1/1(Out1) -> subtract_outbuff1/1
  adder3/1(Out1) -> subtract/2(In2)
  adder2/1(Out1) -> adder1/1(In1)
  square1/1(Out1) -> delayMatch21/1
  subtract/1(Out1) -> subtract_outbuff/1
  adder1/1(Out1) -> adder/1(In1)
  square/1(Out1) -> delayMatch22/1
  adder/1(Out1) -> J/1
  delayMatch8/1 -> subtract6/1(In1)
  subtract_outbuff3/1 -> square3/1(In1), square3/2(In2)
  subtract_outbuff2/1 -> square2/1(In1), square2/2(In2)
  delayMatch20/1 -> adder2/1(In1)
  subtract_outbuff1/1 -> square1/1(In1), square1/2(In2)
  delayMatch21/1 -> adder1/2(In2)
  subtract_outbuff/1 -> square/1(In1), square/2(In2)
  delayMatch22/1 -> adder/2(In2)
  delayMatch19/1 -> subtract/1(In1)
  delayMatch15/1 -> subtract1/1(In1)
  delayMatch11/1 -> subtract2/1(In1)
  delayMatch4/1 -> subtract3/1(In1)
  delayMatch16/1 -> subtract4/1(In1)
  delayMatch12/1 -> subtract5/1(In1)
  delayMatch6/1 -> subtract7/1(In1)
  delayMatch/1 -> subtract8/1(In1)
  delayMatch5/1 -> adder8/1(In1)
  delayMatch7/1 -> multiplier6/1(In1)
  delayMatch18/1 -> adder3/2(In2)
  delayMatch14/1 -> adder4/2(In2)
  delayMatch1/1 -> multiplier7/2(In2)
  delayMatch3/1 -> adder6/2(In2)
  delayMatch17/1 -> multiplier/1(In1)
  delayMatch13/1 -> multiplier1/1(In1)
  delayMatch9/1 -> multiplier3/1(In1)
  delayMatch2/1 -> multiplier4/1(In1)

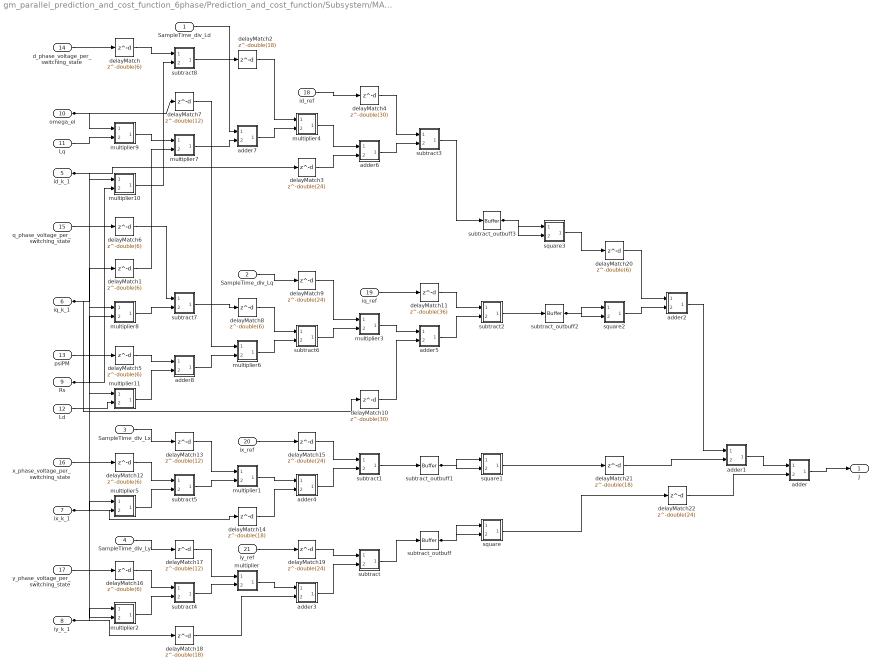
== system gm_parallel_prediction_and_cost_function_6phase/Prediction_and_cost_function/Subsystem/MATLAB Function12 ==
  SampleTime_div_Ld : Inport  OutDataTypeStr=single  PortDimensions=1  SampleTime=1e-08
  SampleTime_div_Lq : Inport  Port=2  OutDataTypeStr=single  PortDimensions=1  SampleTime=1e-08
  SampleTime_div_Lx : Inport  Port=3  OutDataTypeStr=single  PortDimensions=1  SampleTime=1e-08
  SampleTime_div_Ly : Inport  Port=4  OutDataTypeStr=single  PortDimensions=1  SampleTime=1e-08
  id_k_1 : Inport  Port=5  OutDataTypeStr=single  PortDimensions=1  SampleTime=1e-08
  iq_k_1 : Inport  Port=6  OutDataTypeStr=single  PortDimensions=1  SampleTime=1e-08
  ix_k_1 : Inport  Port=7  OutDataTypeStr=single  PortDimensions=1  SampleTime=1e-08
  iy_k_1 : Inport  Port=8  OutDataTypeStr=single  PortDimensions=1  SampleTime=1e-08
  Rs : Inport  Port=9  OutDataTypeStr=single  PortDimensions=1  SampleTime=1e-08
  omega_el : Inport  Port=10  OutDataTypeStr=single  PortDimensions=1  SampleTime=1e-08
  Lq : Inport  Port=11  OutDataTypeStr=single  PortDimensions=1  SampleTime=1e-08
  Ld : Inport  Port=12  OutDataTypeStr=single  PortDimensions=1  SampleTime=1e-08
  psiPM : Inport  Port=13  OutDataTypeStr=single  PortDimensions=1  SampleTime=1e-08
  d_phase_voltage_per_switching_state : Inport  Port=14  OutDataTypeStr=single  PortDimensions=1  SampleTime=1e-08
  q_phase_voltage_per_switching_state : Inport  Port=15  OutDataTypeStr=single  PortDimensions=1  SampleTime=1e-08
  x_phase_voltage_per_switching_state : Inport  Port=16  OutDataTypeStr=single  PortDimensions=1  SampleTime=1e-08
  y_phase_voltage_per_switching_state : Inport  Port=17  OutDataTypeStr=single  PortDimensions=1  SampleTime=1e-08
  id_ref : Inport  Port=18  OutDataTypeStr=single  PortDimensions=1  SampleTime=1e-08
  iq_ref : Inport  Port=19  OutDataTypeStr=single  PortDimensions=1  SampleTime=1e-08
  ix_ref : Inport  Port=20  OutDataTypeStr=single  PortDimensions=1  SampleTime=1e-08
  iy_ref : Inport  Port=21  OutDataTypeStr=single  PortDimensions=1  SampleTime=1e-08
  adder : Subsystem
      mask Display: disp('NFP\nadd');
  adder1 : Subsystem
      mask Display: disp('NFP\nadd');
  adder2 : Subsystem
      mask Display: disp('NFP\nadd');
  adder3 : Subsystem
      mask Display: disp('NFP\nadd');
  adder4 : Subsystem
      mask Display: disp('NFP\nadd');
  adder5 : Subsystem
      mask Display: disp('NFP\nadd');
  adder6 : Subsystem
      mask Display: disp('NFP\nadd');
  adder7 : Subsystem
      mask Display: disp('NFP\nadd');
  adder8 : Subsystem
      mask Display: disp('NFP\nadd');
  delayMatch{,1,5..6,8,12,16,20} (8 alike) : Delay  DelayLength=double(6)  InitialCondition=0  SampleTime=1e-08
  delayMatch10 : Delay  DelayLength=double(30)  InitialCondition=0  SampleTime=1e-08
  delayMatch11 : Delay  DelayLength=double(36)  InitialCondition=0  SampleTime=1e-08
  delayMatch13 : Delay  DelayLength=double(12)  InitialCondition=0  SampleTime=1e-08
  delayMatch{2,14,18,21} (4 alike) : Delay  DelayLength=double(18)  InitialCondition=0  SampleTime=1e-08
  delayMatch{3,9,15,19,22} (5 alike) : Delay  DelayLength=double(24)  InitialCondition=0  SampleTime=1e-08
  delayMatch17 : Delay  DelayLength=double(12)  InitialCondition=0  SampleTime=1e-08
  delayMatch4 : Delay  DelayLength=double(30)  InitialCondition=0  SampleTime=1e-08
  delayMatch7 : Delay  DelayLength=double(12)  InitialCondition=0  SampleTime=1e-08
  multiplier : Subsystem
      mask Display: disp('NFP\nmul');
  multiplier1 : Subsystem
      mask Display: disp('NFP\nmul');
  multiplier10 : Subsystem
      mask Display: disp('NFP\nmul');
  multiplier11 : Subsystem
      mask Display: disp('NFP\nmul');
  multiplier2 : Subsystem
      mask Display: disp('NFP\nmul');
  multiplier3 : Subsystem
      mask Display: disp('NFP\nmul');
  multiplier4 : Subsystem
      mask Display: disp('NFP\nmul');
  multiplier5 : Subsystem
      mask Display: disp('NFP\nmul');
  multiplier6 : Subsystem
      mask Display: disp('NFP\nmul');
  multiplier7 : Subsystem
      mask Display: disp('NFP\nmul');
  multiplier8 : Subsystem
      mask Display: disp('NFP\nmul');
  multiplier9 : Subsystem
      mask Display: disp('NFP\nmul');
  square : Subsystem
      mask Display: disp('NFP\nmul');
  square1 : Subsystem
      mask Display: disp('NFP\nmul');
  square2 : Subsystem
      mask Display: disp('NFP\nmul');
  square3 : Subsystem
      mask Display: disp('NFP\nmul');
  subtract : Subsystem
      mask Display: disp('NFP\nadd');
  subtract1 : Subsystem
      mask Display: disp('NFP\nadd');
  subtract2 : Subsystem
      mask Display: disp('NFP\nadd');
  subtract3 : Subsystem
      mask Display: disp('NFP\nadd');
  subtract4 : Subsystem
      mask Display: disp('NFP\nadd');
  subtract5 : Subsystem
      mask Display: disp('NFP\nadd');
  subtract6 : Subsystem
      mask Display: disp('NFP\nadd');
  subtract7 : Subsystem
      mask Display: disp('NFP\nadd');
  subtract8 : Subsystem
      mask Display: disp('NFP\nadd');
  subtract_outbuff{,1..3} (4 alike) : hdlmdlgenlib/Buffer
      settings: SourceProductBaseCode=SL
  J : Outport  SampleTime=1e-08  VectorParamsAs1DForOutWhenUnconnected=off
  wires:
  iy_ref/1 -> delayMatch19/1
  ix_ref/1 -> delayMatch15/1
  iq_ref/1 -> delayMatch11/1
  id_ref/1 -> delayMatch4/1
  y_phase_voltage_per_switching_state/1 -> delayMatch16/1
  x_phase_voltage_per_switching_state/1 -> delayMatch12/1
  q_phase_voltage_per_switching_state/1 -> delayMatch6/1
  d_phase_voltage_per_switching_state/1 -> delayMatch/1
  psiPM/1 -> delayMatch5/1
  Ld/1 -> multiplier11/2(In2)
  Lq/1 -> multiplier9/2(In2)
  omega_el/1 -> multiplier9/1(In1), delayMatch7/1
  Rs/1 -> multiplier2/2(In2), multiplier5/2(In2), multiplier8/2(In2), multiplier10/2(In2)
  iy_k_1/1 -> multiplier2/1(In1), delayMatch18/1
  ix_k_1/1 -> multiplier5/1(In1), delayMatch14/1
  iq_k_1/1 -> multiplier8/1(In1), delayMatch1/1, delayMatch10/1
  id_k_1/1 -> multiplier10/1(In1), multiplier11/1(In1), delayMatch3/1
  SampleTime_div_Ly/1 -> delayMatch17/1
  SampleTime_div_Lx/1 -> delayMatch13/1
  SampleTime_div_Lq/1 -> delayMatch9/1
  SampleTime_div_Ld/1 -> delayMatch2/1
  delayMatch10/1 -> adder5/2(In2)
  multiplier11/1(Out1) -> adder8/2(In2)
  multiplier10/1(Out1) -> subtract8/2(In2)
  multiplier9/1(Out1) -> multiplier7/1(In1)
  multiplier8/1(Out1) -> subtract7/2(In2)
  adder8/1(Out1) -> multiplier6/2(In2)
  subtract8/1(Out1) -> adder7/1(In1)
  multiplier7/1(Out1) -> adder7/2(In2)
  subtract7/1(Out1) -> delayMatch8/1
  multiplier6/1(Out1) -> subtract6/2(In2)
  adder7/1(Out1) -> multiplier4/2(In2)
  subtract6/1(Out1) -> multiplier3/2(In2)
  multiplier5/1(Out1) -> subtract5/2(In2)
  multiplier4/1(Out1) -> adder6/1(In1)
  multiplier3/1(Out1) -> adder5/1(In1)
  subtract5/1(Out1) -> multiplier1/2(In2)
  multiplier2/1(Out1) -> subtract4/2(In2)
  adder6/1(Out1) -> subtract3/2(In2)
  adder5/1(Out1) -> subtract2/2(In2)
  multiplier1/1(Out1) -> adder4/1(In1)
  subtract4/1(Out1) -> multiplier/2(In2)
  subtract3/1(Out1) -> subtract_outbuff3/1
  subtract2/1(Out1) -> subtract_outbuff2/1
  adder4/1(Out1) -> subtract1/2(In2)
  multiplier/1(Out1) -> adder3/1(In1)
  square3/1(Out1) -> delayMatch20/1
  square2/1(Out1) -> adder2/2(In2)
  subtract1/1(Out1) -> subtract_outbuff1/1
  adder3/1(Out1) -> subtract/2(In2)
  adder2/1(Out1) -> adder1/1(In1)
  square1/1(Out1) -> delayMatch21/1
  subtract/1(Out1) -> subtract_outbuff/1
  adder1/1(Out1) -> adder/1(In1)
  square/1(Out1) -> delayMatch22/1
  adder/1(Out1) -> J/1
  delayMatch8/1 -> subtract6/1(In1)
  subtract_outbuff3/1 -> square3/1(In1), square3/2(In2)
  subtract_outbuff2/1 -> square2/1(In1), square2/2(In2)
  delayMatch20/1 -> adder2/1(In1)
  subtract_outbuff1/1 -> square1/1(In1), square1/2(In2)
  delayMatch21/1 -> adder1/2(In2)
  subtract_outbuff/1 -> square/1(In1), square/2(In2)
  delayMatch22/1 -> adder/2(In2)
  delayMatch19/1 -> subtract/1(In1)
  delayMatch15/1 -> subtract1/1(In1)
  delayMatch11/1 -> subtract2/1(In1)
  delayMatch4/1 -> subtract3/1(In1)
  delayMatch16/1 -> subtract4/1(In1)
  delayMatch12/1 -> subtract5/1(In1)
  delayMatch6/1 -> subtract7/1(In1)
  delayMatch/1 -> subtract8/1(In1)
  delayMatch5/1 -> adder8/1(In1)
  delayMatch7/1 -> multiplier6/1(In1)
  delayMatch18/1 -> adder3/2(In2)
  delayMatch14/1 -> adder4/2(In2)
  delayMatch1/1 -> multiplier7/2(In2)
  delayMatch3/1 -> adder6/2(In2)
  delayMatch17/1 -> multiplier/1(In1)
  delayMatch13/1 -> multiplier1/1(In1)
  delayMatch9/1 -> multiplier3/1(In1)
  delayMatch2/1 -> multiplier4/1(In1)
